simulink model "control_simulink"  (R2020a)
settings: Solver=VariableStepAuto  StartTime=0.0  StopTime=16  RelTol=1e-3
values from neighbouring files (symbols this model uses):
  q = [q,x(:,2:end)]    [CubicPolynomial_viaPoints.m]    (also in HigherOrderPolynomial.m; polynomialtraj.m)
libraries: robotmaniplib x4
settings Model: Creator=Myron Leung  LastModifiedBy=liu_qingzhen

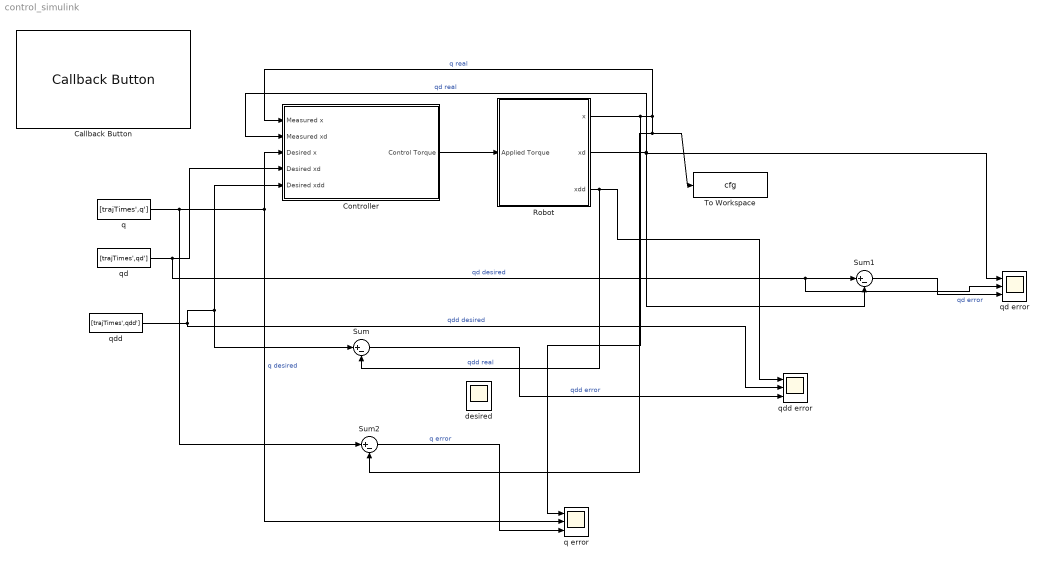
== system control_simulink ==
  Callback Button : CallbackButton  ButtonText=Load_data
      settings: ClickFcn=|
      | clear
      | clc
      | 
      | %%
      | 
      | rootDir = fileparts(which(mfilename));
      | addpath(genpath('matlab'),genpath('simulink'),genpath('utilities'));
      | 
      | load e5
      | 
      | e5waypoints;
      | 
      | eeName='elfin_end_link';
      | numJoints = numel(e5.homeConfiguration);
      | % ikInitGuess = [-1.1829    0.8498    2.3262    0.0000   -1.4764    1.1829];
      | ikInitGuess=[-0.5276    0.7811   -1.7791   -0.0000    2.5600    0.5276];
      | tform = getTransform(e5,ikInitGuess,eeName,'world');
      | endeff=tform2trvec(tform)
      | ik = inverseKinematics('RigidBodyTree',e5);
      | ikWeights = [1 1 1 1 1 1];
      | 
      | 
      | 
      | for idx=1:numel(waypointTimes)
      |     cfg = trvec2tform(waypoints(:,idx)');
      |     [config,info] = ik(eeName,cfg,ikWeights,ikInitGuess);
      | %      ikInitGuess = config;
      |     jointcfg(:,idx)=config';
      | end
      | 
      | %%
      | waypointVels =[0    0.1102    0.2629    0.0890         0;
      |          0    0.0596    0.0884    0.2246         0;
      |          0    0.2625    0.2455    0.2307         0;
      |          0    0.1207    0.1670    0.1413         0;
      |          0    0.0030    0.0484    0.0572         0;
      |          0    0.0971    0.1650    0.0426         0];
      | % waypointVels=[0    0.0532    0.0804    0.0146         0;
      | %           0    0.0465    0.0424    0.0524         0;
      | %           0    0.0277    0.0070    0.0286         0]
      | % 1st
      | 
      | % Acceleration (quintic only)
      | waypointAccels = zeros(size(waypointVels));
      | % 1st      0    0.0532    0.0804    0.0146         0
      | %          0    0.0465    0.0424    0.0524         0
      | %          0    0.0277    0.0070    0.0286         0
      | 
      | %% JOINT SPACE
      | numJoints=6;
      | % [qJoint,qdJoint,qddJoint] = polynomialtraj(jointcfg,waypointTimes,ts);
      | tic
      | traj_type='5th-order Polynomial'
      | switch traj_type
      |     case 'Cubic Polynomial zero'
      |         [q,qd,qdd]=polynomialtraj(jointcfg,waypointTimes,ts);
      |     case '3th-order Polynomial non-zero'
      |         [q,qd,qdd]=CubicPolynomial_viaPoints(jointcfg,waypointVels,waypointTimes,0.1);
      |     case '5th-order Polynomial'
      |         [q,qd,qdd]=HigherOrderPolynomial(jointcfg,waypointVels,waypointAccels,waypointTimes,ts);
      | end
      | jointtime=toc;
      | display(['joint space time ',num2str(jointtime),'s']);
      | 
      | 
      | % plot_joint_trajectory(q);
      | 
      | jointpoints=[]
      | for i =1:size(q,2)
      |     tform=getTransform(e5,q(:,i)',eeName);
      |     jointpoints(:,i)=tform2trvec(tform);
      | end
  Controller : Subsystem
  Robot : Subsystem
  Sum : Sum  Inputs=|+-
  Sum1 : Sum  Inputs=|+-
  Sum2 : Sum  Inputs=|+-
  To Workspace : ToWorkspace  VariableName=cfg  SaveFormat=Timeseries  SampleTime=-1
  desired : Scope
  q : FromWorkspace  VariableName=[trajTimes',q']  SampleTime=0.05
  q error : Scope  NumInputPorts=3
  qd : FromWorkspace  VariableName=[trajTimes',qd']  SampleTime=0.05
  "qd error " : Scope  NumInputPorts=3
  qdd : FromWorkspace  VariableName=[trajTimes',qdd']  SampleTime=0.05
  qdd error : Scope  NumInputPorts=3
  wires:
  Robot/2(xd) -> "qd error "/1, Sum1/2, Controller/2(Measured xd)  "qd real"
  qd/1 -> "qd error "/2, Sum1/1, Controller/4(Desired xd)  "qd desired"
  qdd/1 -> Sum/1, Controller/5(Desired xdd), qdd error/2  "qdd desired"
  Robot/3(xdd) -> Sum/2, qdd error/1  "qdd real"
  Sum1/1 -> "qd error "/3  "qd error"
  q/1 -> Sum2/1, q error/2, Controller/3(Desired x)  "q desired"
  Robot/1(x) -> q error/1, Controller/1(Measured x), To Workspace/1, Sum2/2  "q real"
  Sum2/1 -> q error/3  "q error"
  Controller/1(Control Torque) -> Robot/1(Applied Torque)
  Sum/1 -> qdd error/3  "qdd error"

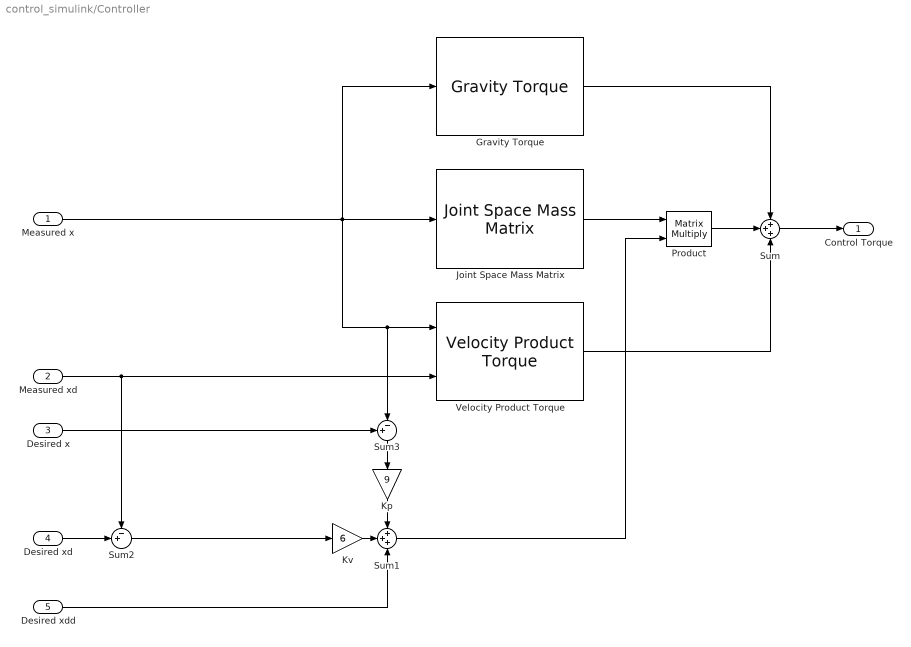
== system control_simulink/Controller ==
  Measured x : Inport
  Measured xd : Inport  Port=2
  Desired x : Inport  Port=3
  Desired xd : Inport  Port=4
  Desired xdd : Inport  Port=5
  Gravity Torque : robotmaniplib/Gravity Torque  RigidBodyTree=e5  SimulateUsing=Interpreted execution
  Joint Space Mass Matrix : robotmaniplib/Joint Space Mass Matrix  RigidBodyTree=e5  SimulateUsing=Interpreted execution
  Kp : Gain  Gain=9
  Kv : Gain  Gain=6
  Product : Product  Multiplication=Matrix(*)
  Sum : Sum  Inputs=+++
  Sum1 : Sum  Inputs=+++
  Sum2 : Sum  Inputs=-+|
  Sum3 : Sum  Inputs=+-|
  Velocity Product Torque : robotmaniplib/Velocity Product Torque  RigidBodyTree=e5  SimulateUsing=Interpreted execution
      settings: SourceProductBaseCode=RO
  Control Torque : Outport
  wires:
  Desired xd/1 -> Sum2/2
  Measured x/1 -> Gravity Torque/1, Joint Space Mass Matrix/1, Sum3/2, Velocity Product Torque/1
  Sum/1 -> Control Torque/1
  Desired x/1 -> Sum3/1
  Sum2/1 -> Kv/1
  Measured xd/1 -> Sum2/1, Velocity Product Torque/2
  Joint Space Mass Matrix/1 -> Product/1
  Kv/1 -> Sum1/2
  Sum1/1 -> Product/2
  Product/1 -> Sum/2
  Sum3/1 -> Kp/1
  Kp/1 -> Sum1/1
  Desired xdd/1 -> Sum1/3
  Gravity Torque/1 -> Sum/1
  Velocity Product Torque/1 -> Sum/3

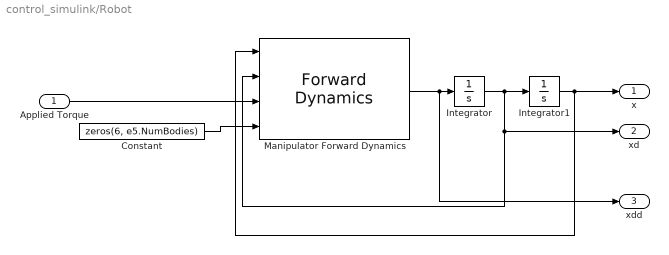
== system control_simulink/Robot ==
  Applied Torque : Inport
  Constant : Constant  Value=zeros(6, e5.NumBodies)
  Integrator : Integrator
  Integrator1 : Integrator  InitialCondition=q(:,1)
  Manipulator Forward Dynamics : robotmaniplib/Forward Dynamics  RigidBodyTree=e5  SimulateUsing=Interpreted execution
  x : Outport
  xd : Outport  Port=2
  xdd : Outport  Port=3
  wires:
  Applied Torque/1 -> Manipulator Forward Dynamics/3
  Integrator/1 -> xd/1, Manipulator Forward Dynamics/2, Integrator1/1
  Manipulator Forward Dynamics/1 -> xdd/1, Integrator/1
  Integrator1/1 -> x/1, Manipulator Forward Dynamics/1
  Constant/1 -> Manipulator Forward Dynamics/4
